simulink model "MIAC_ZTransform_PLC_Coder_not_external_Tustin_test"  (R2018b)
settings: Solver=FixedStepDiscrete  StartTime=0.0  StopTime=60000  FixedStep=1  RelTol=1e-3
libraries: simulink x4, slident x4
(part 1 of 2)
settings Model: Creator=Trips  LastModifiedBy=Trips
settings ConfigComp: PLC_OutputDir=PLCCoder  PLC_TargetIDE=step7  PLC_GenerateReport=off  PLC_LaunchReport=off

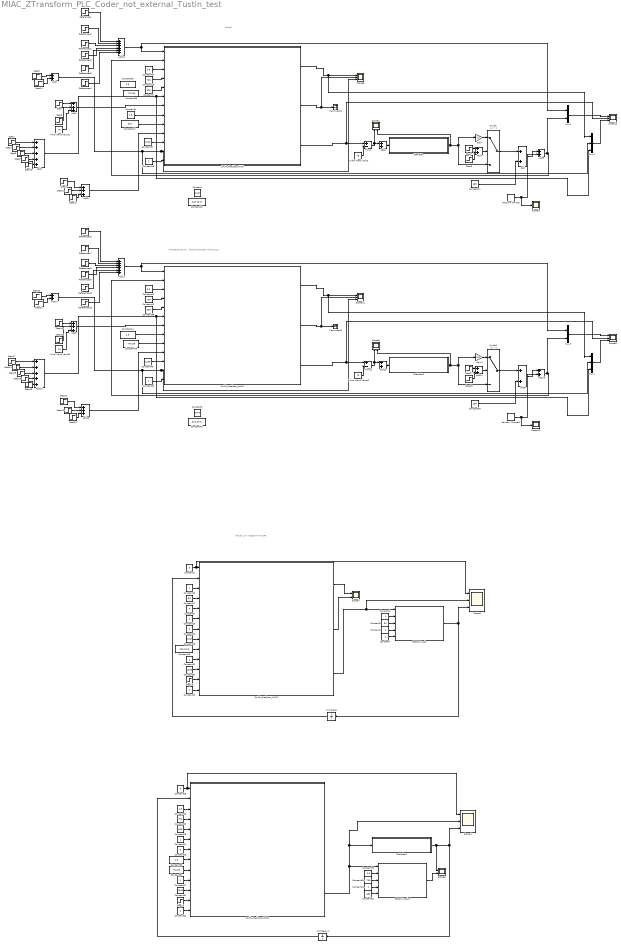
== system MIAC_ZTransform_PLC_Coder_not_external_Tustin_test ==
  note: Mit Adaptivem PI ...funktioniert aber nicht so gut
  note: Aktuell
  note: Aktuell zum vergleich mit SPS
  Add{,3..4,6..8,13..14,16..17} (10 alike) : Sum
  Add{1,5,9,15} (4 alike) : Sum  Inputs=+++
  Add10 : Sum  Inputs=++++++
  Add11 : Sum  Inputs=++++++
  Add12 : Sum  Inputs=5
  Add2 : Sum  Inputs=5
  Constant : Constant  Value=3.047
  Constant{1,28,32,38} (4 alike) : Constant  Value=600
  Constant{4,6,10,13,16,18,21..22,24,27,31,43} (12 alike) : Constant
  Constant11 : Constant  Value=165
  Constant12 : Constant  Value=222.22*3
  Constant{14,19,29,41} (4 alike) : Constant  Value=0.5
  Constant{15,23,30,42} (4 alike) : Constant  Value=700
  Constant17 : Constant  Value=50
  Constant2 : Constant  Value=3
  Constant20 : Constant  Value=0
  Constant25 : Constant  Value=3
  Constant26 : Constant  Value=0
  Constant3 : Constant  Value=5
  Constant33 : Constant  Value=2.5
  Constant34 : Constant  Value=776.39
  Constant35 : Constant  Value=2.5
  Constant36 : Constant  Value=776.39
  Constant{37,46,50..51} (4 alike) : Constant  Value=1200
  Constant39 : Constant  Value=165
  Constant40 : Constant  Value=222.22*3
  Constant44 : Constant  Value=2.5
  Constant45 : Constant  Value=776.39
  Constant47 : Constant  Value=937
  Constant48 : Constant  Value=3.047
  Constant49 : Constant  Value=222.22*3
  Constant5 : Constant  Value=50
  Constant7 : Constant  Value=4
  Constant8 : Constant  Value=1.8
  Constant9 : Constant  Value=3.047
  Drehofen : Subsystem
  Drehofen1 : Subsystem
  Drehofen2 : Subsystem
  FOPDT_Tustin : Subsystem  TreatAsAtomicUnit=on  SystemSampleTime=1
  FOPDT_Tustin1 : Subsystem  TreatAsAtomicUnit=on  SystemSampleTime=1
  Gain : Gain  Gain=1.5
  Gain1 : Gain  Gain=1.5
  Initial Hand Value{,1..3} (4 alike) : Constant  Value=75
  Minus : Sum  Inputs=+-
  Minus1 : Sum  Inputs=+-
  Mux1 : Mux  Inputs=2
  Mux2 : Mux  Inputs=3
  Mux3 : Mux  Inputs=2
  Mux4 : Mux  Inputs=3
  Random Number : RandomNumber  Variance=0.01  SampleTime=10
  Random Number1 : RandomNumber  Variance=0.01  SampleTime=10
  References : Step  After=3
  References1 : Step  Time=12000  After=2
  References10 : Step  Time=0  After=165
  References11 : Step  Time=40000  After=-7
  References2 : Step  Time=18000  After=3
  References3 : Step  Time=35000  After=3
  References4 : Step  Time=0  After=165
  References5 : Step  Time=40000  After=-7
  References6 : Step  After=3
  References7 : Step  Time=12000  After=2
  References8 : Step  Time=18000  After=3
  References9 : Step  Time=35000  After=3
  Scope{1,5,7..8} (4 alike) : Scope  NumInputPorts=2
  Scope10 : Scope
  Scope{2,4,6,9,11..12} (6 alike) : Scope  NumInputPorts=3
  Scope3 : Scope
  Smith_Predictor_MIAC : Subsystem  TreatAsAtomicUnit=on  SystemSampleTime=1
  Smith_Predictor_MIAC1 : Subsystem  TreatAsAtomicUnit=on  SystemSampleTime=1
  Smith_Predictor_MIAC2 : Subsystem  TreatAsAtomicUnit=on  SystemSampleTime=1
  Smith_Predictor_MIAC4 : Subsystem  TreatAsAtomicUnit=on  SystemSampleTime=1
  Step : Step  Time=300  After=5  SampleTime=0
  Step1 : Step  Time=4000  SampleTime=0
  Step10 : Step  Time=50000  SampleTime=0
  Step11 : Step  Time=35000  After=-1  SampleTime=0
  Step12 : Step  Time=38000  SampleTime=1
  Step13 : Step  Time=500  After=0  SampleTime=0
  Step14 : Step  Time=2.5*10^4  SampleTime=1
  Step15 : Step  Time=500  After=0  SampleTime=0
  Step16 : Step  Time=300  After=5  SampleTime=0
  Step17 : Step  Time=4000  SampleTime=0
  Step18 : Step  Time=50000  SampleTime=0
  Step19 : Step  Time=35000  After=-1  SampleTime=0
  Step2 : Step  Time=3900  SampleTime=1
  Step20 : Step  Time=38000  SampleTime=1
  Step21 : Step  Time=2.5*10^4  SampleTime=1
  Step22 : Step  Time=3900  SampleTime=1
  Step23 : Step  Time=5000  Before=1  After=0  SampleTime=1
  Step24 : Step  Time=20000  After=-1  SampleTime=0
  Step25 : Step  Time=25000  SampleTime=0
  Step26 : Step  Time=19000  After=5  SampleTime=0
  Step27 : Step  Time=3*10^4  SampleTime=0
  Step28 : Step  Time=3.8*10^4  After=0  SampleTime=0
  Step29 : Step  Time=45000  After=-1  SampleTime=0
  Step3 : Step  Time=5000  Before=1  After=0  SampleTime=1
  Step4 : Step  Time=20000  After=-1  SampleTime=0
  Step5 : Step  Time=25000  SampleTime=0
  Step6 : Step  Time=19000  After=5  SampleTime=0
  Step7 : Step  Time=3*10^4  SampleTime=0
  Step8 : Step  Time=3.8*10^4  After=0  SampleTime=0
  Step9 : Step  Time=45000  After=-1  SampleTime=0
  Switch : Switch  Criteria=u2 > Threshold
  Switch1 : Switch  Criteria=u2 > Threshold
  Terminator1 : Terminator
  Terminator2 : Terminator
  Unit Delay : UnitDelay  SampleTime=-1
  Unit Delay1 : UnitDelay  SampleTime=-1
  wires:
  Smith_Predictor_MIAC/1(Gain_NOT_Filtered) -> Mux2/1, Scope6/1  "Gain Filtered"
  Smith_Predictor_MIAC/2(Gain_Filtered) -> Scope6/2, Terminator1/1
  Add10/1 -> Mux1/1, Smith_Predictor_MIAC/1(Setpoint)  "setpoint"
  Step8/1 -> Add4/2
  Smith_Predictor_MIAC/3(Controller_Value) -> Scope12/2, Minus/1  "Adaptive"
  Add4/1 -> Switch/2  "Fehler ein"
  Gain/1 -> Switch/1
  Minus/1 -> Add6/1, Scope1/1
  Add6/1 -> Drehofen/1(In1)
  Drehofen/1(Out1) -> Scope1/2, Gain/1, Switch/3
  Step7/1 -> Add4/1
  Random Number/1 -> Scope3/1, Add3/2
  Initial Hand Value/1 -> Minus/2
  Add/1 -> Add3/1  "MIAC_SmithPredictor"
  Switch/1 -> Add/1  "MIAC_SmithPredictor"
  Constant11/1 -> Add/2
  Add3/1 -> Mux1/2, Smith_Predictor_MIAC/2(Process_Value)  "MIAC_SmithPredictor"
  References3/1 -> Add10/4  "r"
  References/1 -> Add10/1  "r"
  References4/1 -> Add10/6  "r"
  References1/1 -> Add10/2  "r"
  References2/1 -> Add10/3  "r"
  References5/1 -> Add10/5
  Constant8/1 -> Smith_Predictor_MIAC/8(P_Controller)
  Constant47/1 -> Smith_Predictor_MIAC/9(I_Controller)
  Constant14/1 -> Smith_Predictor_MIAC/3(Gain_System)
  Constant15/1 -> Smith_Predictor_MIAC/4(Time_Constant_System)
  Constant16/1 -> Smith_Predictor_MIAC/13(Sample_Time)
  Constant1/1 -> Smith_Predictor_MIAC/5(Dead_Time_System)
  Step14/1 -> Add7/2  "Start Adaption"
  Step3/1 -> Add7/1  "Start Adaption"
  Add7/1 -> Mux2/2, Scope6/3, Smith_Predictor_MIAC/12(Enable_Adaption)  "Start Adaption"
  Step6/1 -> Add1/2
  Initial Hand Value1/1 -> Add1/3
  Step/1 -> Add1/1
  Add1/1 -> Smith_Predictor_MIAC/7(Hand_Value)
  Step9/1 -> Add2/4  "Einschalten Automatik"
  Step10/1 -> Add2/5  "Einschalten Automatik"
  Step5/1 -> Add2/3  "Einschalten Automatik"
  Step4/1 -> Add2/2  "Einschalten Automatik"
  Step1/1 -> Add2/1  "Einschalten Automatik"
  Add2/1 -> Mux2/3, Smith_Predictor_MIAC/6(" Enable_Auto")  "Einschalten Automatik"
  Step12/1 -> Add5/3  "Start Identification"
  Step11/1 -> Add5/2  "Einschalten Automatik"
  Step2/1 -> Add5/1  "Start Identification"
  Add5/1 -> Smith_Predictor_MIAC/10(Start_Identification)  "Start Identification"
  Constant6/1 -> FOPDT_Tustin/4(Sample_Time)
  Constant17/1 -> Smith_Predictor_MIAC1/4(Time_Constant_System)
  Constant21/1 -> Smith_Predictor_MIAC1/10(Start_Identification)
  Constant10/1 -> Smith_Predictor_MIAC1/3(Gain_System)
  Constant49/1 -> Smith_Predictor_MIAC1/9(I_Controller)
  Constant18/1 -> Smith_Predictor_MIAC1/6(" Enable_Auto")
  Constant48/1 -> Smith_Predictor_MIAC1/8(P_Controller)
  Constant7/1 -> FOPDT_Tustin/5(" Dead_Time")
  Constant4/1 -> FOPDT_Tustin/2(Gain_System)
  Constant20/1 -> Smith_Predictor_MIAC1/7(Hand_Value)
  Constant2/1 -> Smith_Predictor_MIAC1/1(Setpoint), Scope2/1
  Constant5/1 -> FOPDT_Tustin/3(Time_Constant_System)
  Constant3/1 -> Smith_Predictor_MIAC1/5(Dead_Time_System)
  Smith_Predictor_MIAC1/3(Controller_Value) -> Scope2/2, FOPDT_Tustin/1(FOPD_Input)  "Adaptive"
  FOPDT_Tustin/1(FOPD_Output) -> Unit Delay/1, Scope2/3  "tustin"
  Unit Delay/1 -> Smith_Predictor_MIAC1/2(Process_Value)
  Unit Delay1/1 -> Smith_Predictor_MIAC2/2(Process_Value)
  Constant22/1 -> Smith_Predictor_MIAC2/13(Sample_Time)
  Drehofen1/1(Out1) -> Scope5/1, Scope4/3, Unit Delay1/1
  Constant26/1 -> Smith_Predictor_MIAC2/7(Hand_Value)
  Constant34/1 -> Smith_Predictor_MIAC2/9(I_Controller)
  Constant19/1 -> Smith_Predictor_MIAC2/3(Gain_System)
  Constant28/1 -> Smith_Predictor_MIAC2/5(Dead_Time_System)
  Constant33/1 -> Smith_Predictor_MIAC2/8(P_Controller)
  Constant27/1 -> Smith_Predictor_MIAC2/10(Start_Identification)
  Constant25/1 -> Smith_Predictor_MIAC2/1(Setpoint), Scope4/1
  Constant23/1 -> Smith_Predictor_MIAC2/4(Time_Constant_System)
  Constant24/1 -> Smith_Predictor_MIAC2/6(" Enable_Auto")
  Step15/1 -> Smith_Predictor_MIAC2/12(Enable_Adaption)
  Smith_Predictor_MIAC2/3(Controller_Value) -> FOPDT_Tustin1/1(FOPD_Input), Drehofen1/1(In1), Scope4/2  "Adaptive"
  Constant29/1 -> FOPDT_Tustin1/2(Gain_System)
  Constant31/1 -> FOPDT_Tustin1/4(Sample_Time)
  Constant30/1 -> FOPDT_Tustin1/3(Time_Constant_System)
  Constant32/1 -> FOPDT_Tustin1/5(" Dead_Time")
  FOPDT_Tustin1/1(FOPD_Output) -> Scope5/2  "tustin"
  Smith_Predictor_MIAC1/1(Gain_NOT_Filtered) -> Scope7/1  "Gain Filtered"
  Smith_Predictor_MIAC1/2(Gain_Filtered) -> Scope7/2
  Constant37/1 -> Smith_Predictor_MIAC/11(Time_Constant_Gain_identification_Filter)
  Mux1/1 -> Scope12/1
  Mux2/1 -> Scope12/3
  Mux3/1 -> Scope9/1
  Step20/1 -> Add15/3  "Start Identification"
  Step17/1 -> Add12/1  "Einschalten Automatik"
  Step25/1 -> Add12/3  "Einschalten Automatik"
  Step24/1 -> Add12/2  "Einschalten Automatik"
  References9/1 -> Add11/4  "r"
  Step19/1 -> Add15/2  "Einschalten Automatik"
  Step21/1 -> Add17/2  "Start Adaption"
  Step23/1 -> Add17/1  "Start Adaption"
  Add11/1 -> Mux3/1, Smith_Predictor_MIAC4/1(Setpoint)  "setpoint"
  References10/1 -> Add11/6  "r"
  Step29/1 -> Add12/4  "Einschalten Automatik"
  Add13/1 -> Mux3/2, Smith_Predictor_MIAC4/2(Process_Value)  "MIAC_SmithPredictor"
  Constant39/1 -> Add8/2
  Gain1/1 -> Switch1/1
  Random Number1/1 -> Scope10/1, Add13/2
  Initial Hand Value3/1 -> Add9/3
  Add16/1 -> Drehofen2/1(In1)
  Drehofen2/1(Out1) -> Scope8/2, Gain1/1, Switch1/3
  Step18/1 -> Add12/5  "Einschalten Automatik"
  Constant46/1 -> Smith_Predictor_MIAC4/11(Time_Constant_Gain_identification_Filter)
  Switch1/1 -> Add8/1  "MIAC_SmithPredictor"
  Constant43/1 -> Smith_Predictor_MIAC4/13(Sample_Time)
  Step28/1 -> Add14/2
  Smith_Predictor_MIAC4/2(Gain_Filtered) -> Scope11/2, Terminator2/1
  Constant44/1 -> Smith_Predictor_MIAC4/8(P_Controller)
  Step27/1 -> Add14/1
  Add15/1 -> Smith_Predictor_MIAC4/10(Start_Identification)  "Start Identification"
  Add17/1 -> Mux4/2, Scope11/3, Smith_Predictor_MIAC4/12(Enable_Adaption)  "Start Adaption"
  Constant45/1 -> Smith_Predictor_MIAC4/9(I_Controller)
  Mux4/1 -> Scope9/3
  Smith_Predictor_MIAC4/1(Gain_NOT_Filtered) -> Mux4/1, Scope11/1  "Gain Filtered"
  Initial Hand Value2/1 -> Minus1/2
  Add14/1 -> Switch1/2  "Fehler ein"
  Smith_Predictor_MIAC4/3(Controller_Value) -> Scope9/2, Minus1/1  "Adaptive"
  References11/1 -> Add11/5
  Constant41/1 -> Smith_Predictor_MIAC4/3(Gain_System)
  References7/1 -> Add11/2  "r"
  Add9/1 -> Smith_Predictor_MIAC4/7(Hand_Value)
  References6/1 -> Add11/1  "r"
  Step16/1 -> Add9/1
  Step22/1 -> Add15/1  "Start Identification"
  Add8/1 -> Add13/1  "MIAC_SmithPredictor"
  Add12/1 -> Mux4/3, Smith_Predictor_MIAC4/6(" Enable_Auto")  "Einschalten Automatik"
  Constant42/1 -> Smith_Predictor_MIAC4/4(Time_Constant_System)
  References8/1 -> Add11/3  "r"
  Minus1/1 -> Add16/1, Scope8/1
  Constant38/1 -> Smith_Predictor_MIAC4/5(Dead_Time_System)
  Step26/1 -> Add9/2
  Step13/1 -> Smith_Predictor_MIAC1/12(Enable_Adaption)
  Constant13/1 -> Smith_Predictor_MIAC1/13(Sample_Time)
  Constant50/1 -> Smith_Predictor_MIAC1/11(Time_Constant_Gain_identification_Filter)
  Constant51/1 -> Smith_Predictor_MIAC2/11(Time_Constant_Gain_identification_Filter)

== system MIAC_ZTransform_PLC_Coder_not_external_Tustin_test/Drehofen ==
  In1 : Inport
  Constant3 : Constant  Value=0.5/700
  Constant4 : Constant  Value=[1 -exp(-1/700)]
  Delay : Delay  DelayLength=600
  Discrete Transfer Fcn : DiscreteTransferFcn  NumeratorSource=Input port  DenominatorSource=Input port  a0EqualsOne=on
      settings: InputPortMap=u0,p1,p3
  Out1 : Outport
  wires:
  Discrete Transfer Fcn/1 -> Delay/1
  Constant4/1 -> Discrete Transfer Fcn/3
  Constant3/1 -> Discrete Transfer Fcn/2
  In1/1 -> Discrete Transfer Fcn/1
  Delay/1 -> Out1/1  "MIAC_SmithPredictor"

== system MIAC_ZTransform_PLC_Coder_not_external_Tustin_test/Drehofen1 ==
  In1 : Inport
  Constant3 : Constant  Value=0.5/700
  Constant4 : Constant  Value=[1 -exp(-1/700)]
  Delay : Delay  DelayLength=600
  Discrete Transfer Fcn : DiscreteTransferFcn  NumeratorSource=Input port  DenominatorSource=Input port  a0EqualsOne=on
      settings: InputPortMap=u0,p1,p3
  Out1 : Outport
  wires:
  Discrete Transfer Fcn/1 -> Delay/1
  Constant4/1 -> Discrete Transfer Fcn/3
  Constant3/1 -> Discrete Transfer Fcn/2
  In1/1 -> Discrete Transfer Fcn/1
  Delay/1 -> Out1/1  "MIAC_SmithPredictor"

== system MIAC_ZTransform_PLC_Coder_not_external_Tustin_test/Drehofen2 ==
  In1 : Inport
  Constant3 : Constant  Value=0.5/700
  Constant4 : Constant  Value=[1 -exp(-1/700)]
  Delay : Delay  DelayLength=600
  Discrete Transfer Fcn : DiscreteTransferFcn  NumeratorSource=Input port  DenominatorSource=Input port  a0EqualsOne=on
      settings: InputPortMap=u0,p1,p3
  Out1 : Outport
  wires:
  Discrete Transfer Fcn/1 -> Delay/1
  Constant4/1 -> Discrete Transfer Fcn/3
  Constant3/1 -> Discrete Transfer Fcn/2
  In1/1 -> Discrete Transfer Fcn/1
  Delay/1 -> Out1/1  "MIAC_SmithPredictor"

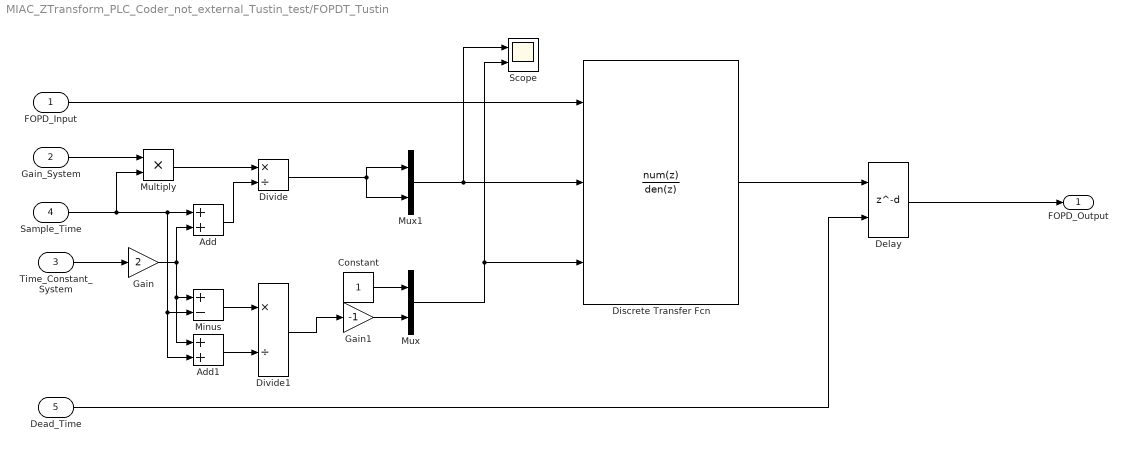
== system MIAC_ZTransform_PLC_Coder_not_external_Tustin_test/FOPDT_Tustin ==
  FOPD_Input : Inport
  Gain_System : Inport  Port=2
  Time_Constant_System : Inport  Port=3
  Sample_Time : Inport  Port=4
  " Dead_Time" : Inport  Port=5
  Add : Sum
  Add1 : Sum
  Constant : Constant
  Delay : Delay  DelayLengthSource=Input port  DelayLength=600  DelayLengthUpperLimit=800
      settings: InputPortMap=u0,p1
  Discrete Transfer Fcn : DiscreteTransferFcn  NumeratorSource=Input port  DenominatorSource=Input port  SampleTime=1  a0EqualsOne=on
      settings: InputPortMap=u0,p1,p3
  Divide : Product  Inputs=*/
  Divide1 : Product  Inputs=*/
  Gain : Gain  Gain=2
  Gain1 : Gain  Gain=-1
  Minus : Sum  Inputs=+-
  Multiply : Product
  Mux : Mux  Inputs=2
  Mux1 : Mux  Inputs=2
  Scope : Scope  NumInputPorts=2
  FOPD_Output : Outport
  wires:
  FOPD_Input/1 -> Discrete Transfer Fcn/1
  Discrete Transfer Fcn/1 -> Delay/1
  Mux/1 -> Scope/2, Discrete Transfer Fcn/3
  " Dead_Time"/1 -> Delay/2
  Sample_Time/1 -> Add1/2, Minus/2, Add/1, Multiply/2
  Mux1/1 -> Scope/1, Discrete Transfer Fcn/2
  Time_Constant_System/1 -> Gain/1
  Delay/1 -> FOPD_Output/1
  Gain_System/1 -> Multiply/1
  Multiply/1 -> Divide/1
  Gain/1 -> Add1/1, Minus/1, Add/2
  Add/1 -> Divide/2
  Divide/1 -> Mux1/2, Mux1/1
  Constant/1 -> Mux/1
  Minus/1 -> Divide1/1
  Add1/1 -> Divide1/2
  Divide1/1 -> Gain1/1
  Gain1/1 -> Mux/2

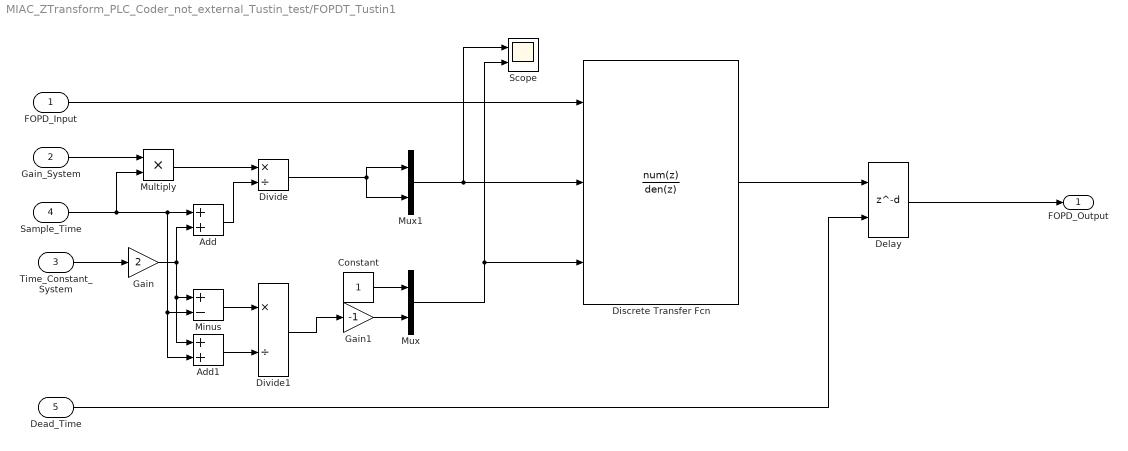
== system MIAC_ZTransform_PLC_Coder_not_external_Tustin_test/FOPDT_Tustin1 ==
  FOPD_Input : Inport
  Gain_System : Inport  Port=2
  Time_Constant_System : Inport  Port=3
  Sample_Time : Inport  Port=4
  " Dead_Time" : Inport  Port=5
  Add : Sum
  Add1 : Sum
  Constant : Constant
  Delay : Delay  DelayLengthSource=Input port  DelayLength=600  DelayLengthUpperLimit=800
      settings: InputPortMap=u0,p1
  Discrete Transfer Fcn : DiscreteTransferFcn  NumeratorSource=Input port  DenominatorSource=Input port  SampleTime=1  a0EqualsOne=on
      settings: InputPortMap=u0,p1,p3
  Divide : Product  Inputs=*/
  Divide1 : Product  Inputs=*/
  Gain : Gain  Gain=2
  Gain1 : Gain  Gain=-1
  Minus : Sum  Inputs=+-
  Multiply : Product
  Mux : Mux  Inputs=2
  Mux1 : Mux  Inputs=2
  Scope : Scope  NumInputPorts=2
  FOPD_Output : Outport
  wires:
  FOPD_Input/1 -> Discrete Transfer Fcn/1
  Discrete Transfer Fcn/1 -> Delay/1
  Mux/1 -> Scope/2, Discrete Transfer Fcn/3
  " Dead_Time"/1 -> Delay/2
  Sample_Time/1 -> Add1/2, Minus/2, Add/1, Multiply/2
  Mux1/1 -> Scope/1, Discrete Transfer Fcn/2
  Time_Constant_System/1 -> Gain/1
  Delay/1 -> FOPD_Output/1
  Gain_System/1 -> Multiply/1
  Multiply/1 -> Divide/1
  Gain/1 -> Add1/1, Minus/1, Add/2
  Add/1 -> Divide/2
  Divide/1 -> Mux1/2, Mux1/1
  Constant/1 -> Mux/1
  Minus/1 -> Divide1/1
  Add1/1 -> Divide1/2
  Divide1/1 -> Gain1/1
  Gain1/1 -> Mux/2

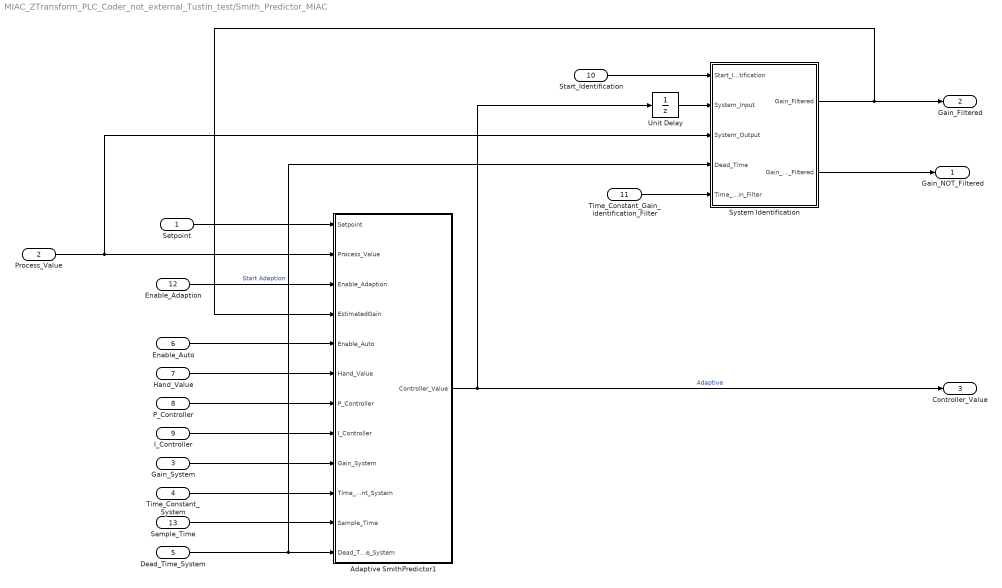
== system MIAC_ZTransform_PLC_Coder_not_external_Tustin_test/Smith_Predictor_MIAC ==
  Setpoint : Inport
  Process_Value : Inport  Port=2
  Gain_System : Inport  Port=3
  Time_Constant_System : Inport  Port=4
  Dead_Time_System : Inport  Port=5
  " Enable_Auto" : Inport  Port=6
  Hand_Value : Inport  Port=7
  P_Controller : Inport  Port=8
  I_Controller : Inport  Port=9
  Start_Identification : Inport  Port=10  PortDimensions=1  SampleTime=1
  Time_Constant_Gain_identification_Filter : Inport  Port=11
  Enable_Adaption : Inport  Port=12
  Sample_Time : Inport  Port=13
  Adaptive SmithPredictor1 : Subsystem  TreatAsAtomicUnit=on  SystemSampleTime=1
  System Identification : Subsystem  TreatAsAtomicUnit=on  SystemSampleTime=1
  Unit Delay : UnitDelay
  Gain_NOT_Filtered : Outport
  Gain_Filtered : Outport  Port=2
  Controller_Value : Outport  Port=3
  wires:
  Gain_System/1 -> Adaptive SmithPredictor1/9(Gain_System)
  Dead_Time_System/1 -> Adaptive SmithPredictor1/12(" Dead_Time_System"), System Identification/4(Dead_Time)
  Adaptive SmithPredictor1/1(Controller_Value) -> Unit Delay/1, Controller_Value/1  "Adaptive"
  Time_Constant_System/1 -> Adaptive SmithPredictor1/10(Time_Constant_System)
  P_Controller/1 -> Adaptive SmithPredictor1/7(P_Controller)
  Sample_Time/1 -> Adaptive SmithPredictor1/11(Sample_Time)
  I_Controller/1 -> Adaptive SmithPredictor1/8(I_Controller)
  Enable_Adaption/1 -> Adaptive SmithPredictor1/3(Enable_Adaption)  "Start Adaption"
  System Identification/2(Gain_Not_Filtered) -> Gain_NOT_Filtered/1
  Setpoint/1 -> Adaptive SmithPredictor1/1(Setpoint)
  Start_Identification/1 -> System Identification/1(Start_Identification)
  System Identification/1(Gain_Filtered) -> Gain_Filtered/1, Adaptive SmithPredictor1/4(EstimatedGain)
  " Enable_Auto"/1 -> Adaptive SmithPredictor1/5(Enable_Auto)
  Hand_Value/1 -> Adaptive SmithPredictor1/6(Hand_Value)
  Process_Value/1 -> System Identification/3(System_Output), Adaptive SmithPredictor1/2(Process_Value)
  Unit Delay/1 -> System Identification/2(System_Input)
  Time_Constant_Gain_identification_Filter/1 -> System Identification/5(Time_Constant_Gain_Filter)

== system MIAC_ZTransform_PLC_Coder_not_external_Tustin_test/Smith_Predictor_MIAC1 ==
  Setpoint : Inport
  Process_Value : Inport  Port=2
  Gain_System : Inport  Port=3
  Time_Constant_System : Inport  Port=4
  Dead_Time_System : Inport  Port=5
  " Enable_Auto" : Inport  Port=6
  Hand_Value : Inport  Port=7
  P_Controller : Inport  Port=8
  I_Controller : Inport  Port=9
  Start_Identification : Inport  Port=10  PortDimensions=1  SampleTime=1
  Time_Constant_Gain_identification_Filter : Inport  Port=11
  Enable_Adaption : Inport  Port=12
  Sample_Time : Inport  Port=13
  Adaptive SmithPredictor1 : Subsystem  TreatAsAtomicUnit=on  SystemSampleTime=1
  System Identification : Subsystem  TreatAsAtomicUnit=on  SystemSampleTime=1
  Unit Delay : UnitDelay
  Gain_NOT_Filtered : Outport
  Gain_Filtered : Outport  Port=2
  Controller_Value : Outport  Port=3
  wires:
  Gain_System/1 -> Adaptive SmithPredictor1/9(Gain_System)
  Dead_Time_System/1 -> Adaptive SmithPredictor1/12(" Dead_Time_System"), System Identification/4(Dead_Time)
  Adaptive SmithPredictor1/1(Controller_Value) -> Unit Delay/1, Controller_Value/1  "Adaptive"
  Time_Constant_System/1 -> Adaptive SmithPredictor1/10(Time_Constant_System)
  P_Controller/1 -> Adaptive SmithPredictor1/7(P_Controller)
  Sample_Time/1 -> Adaptive SmithPredictor1/11(Sample_Time)
  I_Controller/1 -> Adaptive SmithPredictor1/8(I_Controller)
  Enable_Adaption/1 -> Adaptive SmithPredictor1/3(Enable_Adaption)  "Start Adaption"
  System Identification/2(Gain_Not_Filtered) -> Gain_NOT_Filtered/1
  Setpoint/1 -> Adaptive SmithPredictor1/1(Setpoint)
  Start_Identification/1 -> System Identification/1(Start_Identification)
  System Identification/1(Gain_Filtered) -> Gain_Filtered/1, Adaptive SmithPredictor1/4(EstimatedGain)
  " Enable_Auto"/1 -> Adaptive SmithPredictor1/5(Enable_Auto)
  Hand_Value/1 -> Adaptive SmithPredictor1/6(Hand_Value)
  Process_Value/1 -> System Identification/3(System_Output), Adaptive SmithPredictor1/2(Process_Value)
  Unit Delay/1 -> System Identification/2(System_Input)
  Time_Constant_Gain_identification_Filter/1 -> System Identification/5(Time_Constant_Gain_Filter)

== system MIAC_ZTransform_PLC_Coder_not_external_Tustin_test/Smith_Predictor_MIAC2 ==
  Setpoint : Inport
  Process_Value : Inport  Port=2
  Gain_System : Inport  Port=3
  Time_Constant_System : Inport  Port=4
  Dead_Time_System : Inport  Port=5
  " Enable_Auto" : Inport  Port=6
  Hand_Value : Inport  Port=7
  P_Controller : Inport  Port=8
  I_Controller : Inport  Port=9
  Start_Identification : Inport  Port=10  PortDimensions=1  SampleTime=1
  Time_Constant_Gain_identification_Filter : Inport  Port=11
  Enable_Adaption : Inport  Port=12
  Sample_Time : Inport  Port=13
  Adaptive SmithPredictor1 : Subsystem  TreatAsAtomicUnit=on  SystemSampleTime=1
  System Identification : Subsystem  TreatAsAtomicUnit=on  SystemSampleTime=1
  Unit Delay : UnitDelay
  Gain_NOT_Filtered : Outport
  Gain_Filtered : Outport  Port=2
  Controller_Value : Outport  Port=3
  wires:
  Gain_System/1 -> Adaptive SmithPredictor1/9(Gain_System)
  Dead_Time_System/1 -> Adaptive SmithPredictor1/12(" Dead_Time_System"), System Identification/4(Dead_Time)
  Adaptive SmithPredictor1/1(Controller_Value) -> Unit Delay/1, Controller_Value/1  "Adaptive"
  Time_Constant_System/1 -> Adaptive SmithPredictor1/10(Time_Constant_System)
  P_Controller/1 -> Adaptive SmithPredictor1/7(P_Controller)
  Sample_Time/1 -> Adaptive SmithPredictor1/11(Sample_Time)
  I_Controller/1 -> Adaptive SmithPredictor1/8(I_Controller)
  Enable_Adaption/1 -> Adaptive SmithPredictor1/3(Enable_Adaption)  "Start Adaption"
  System Identification/2(Gain_Not_Filtered) -> Gain_NOT_Filtered/1
  Setpoint/1 -> Adaptive SmithPredictor1/1(Setpoint)
  Start_Identification/1 -> System Identification/1(Start_Identification)
  System Identification/1(Gain_Filtered) -> Gain_Filtered/1, Adaptive SmithPredictor1/4(EstimatedGain)
  " Enable_Auto"/1 -> Adaptive SmithPredictor1/5(Enable_Auto)
  Hand_Value/1 -> Adaptive SmithPredictor1/6(Hand_Value)
  Process_Value/1 -> System Identification/3(System_Output), Adaptive SmithPredictor1/2(Process_Value)
  Unit Delay/1 -> System Identification/2(System_Input)
  Time_Constant_Gain_identification_Filter/1 -> System Identification/5(Time_Constant_Gain_Filter)

== system MIAC_ZTransform_PLC_Coder_not_external_Tustin_test/Smith_Predictor_MIAC4 ==
  Setpoint : Inport
  Process_Value : Inport  Port=2
  Gain_System : Inport  Port=3
  Time_Constant_System : Inport  Port=4
  Dead_Time_System : Inport  Port=5
  " Enable_Auto" : Inport  Port=6
  Hand_Value : Inport  Port=7
  P_Controller : Inport  Port=8
  I_Controller : Inport  Port=9
  Start_Identification : Inport  Port=10  PortDimensions=1  SampleTime=1
  Time_Constant_Gain_identification_Filter : Inport  Port=11
  Enable_Adaption : Inport  Port=12
  Sample_Time : Inport  Port=13
  Adaptive SmithPredictor1 : Subsystem  TreatAsAtomicUnit=on  SystemSampleTime=1
  System Identification : Subsystem  TreatAsAtomicUnit=on  SystemSampleTime=1
  Unit Delay : UnitDelay
  Gain_NOT_Filtered : Outport
  Gain_Filtered : Outport  Port=2
  Controller_Value : Outport  Port=3
  wires:
  Gain_System/1 -> Adaptive SmithPredictor1/9(Gain_System)
  Dead_Time_System/1 -> Adaptive SmithPredictor1/12(" Dead_Time_System"), System Identification/4(Dead_Time)
  Adaptive SmithPredictor1/1(Controller_Value) -> Unit Delay/1, Controller_Value/1  "Adaptive"
  Time_Constant_System/1 -> Adaptive SmithPredictor1/10(Time_Constant_System)
  P_Controller/1 -> Adaptive SmithPredictor1/7(P_Controller)
  Sample_Time/1 -> Adaptive SmithPredictor1/11(Sample_Time)
  I_Controller/1 -> Adaptive SmithPredictor1/8(I_Controller)
  Enable_Adaption/1 -> Adaptive SmithPredictor1/3(Enable_Adaption)  "Start Adaption"
  System Identification/2(Gain_Not_Filtered) -> Gain_NOT_Filtered/1
  Setpoint/1 -> Adaptive SmithPredictor1/1(Setpoint)
  Start_Identification/1 -> System Identification/1(Start_Identification)
  System Identification/1(Gain_Filtered) -> Gain_Filtered/1, Adaptive SmithPredictor1/4(EstimatedGain)
  " Enable_Auto"/1 -> Adaptive SmithPredictor1/5(Enable_Auto)
  Hand_Value/1 -> Adaptive SmithPredictor1/6(Hand_Value)
  Process_Value/1 -> System Identification/3(System_Output), Adaptive SmithPredictor1/2(Process_Value)
  Unit Delay/1 -> System Identification/2(System_Input)
  Time_Constant_Gain_identification_Filter/1 -> System Identification/5(Time_Constant_Gain_Filter)

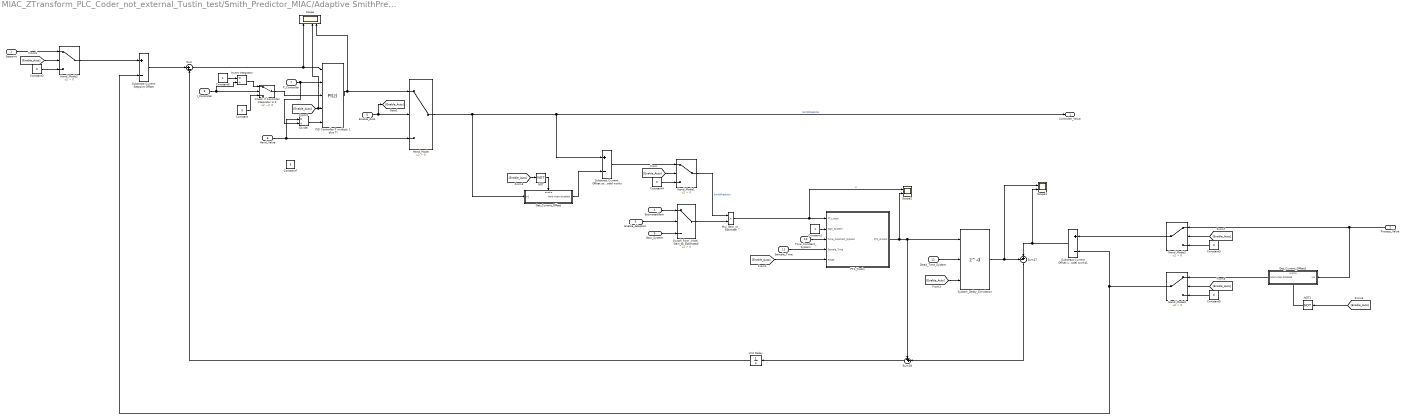
== system MIAC_ZTransform_PLC_Coder_not_external_Tustin_test/Smith_Predictor_MIAC/Adaptive SmithPredictor1 ==
  Setpoint : Inport
  Process_Value : Inport  Port=2
  Enable_Adaption : Inport  Port=3
  EstimatedGain : Inport  Port=4
  Enable_Auto : Inport  Port=5
  Hand_Value : Inport  Port=6
  P_Controller : Inport  Port=7
  I_Controller : Inport  Port=8
  Gain_System : Inport  Port=9
  Time_Constant_System : Inport  Port=10
  Sample_Time : Inport  Port=11
  " Dead_Time_System" : Inport  Port=12
  Check if Controller Integrator is 0 : Switch  Criteria=u2 ~= 0
  Constant{,2..5} (5 alike) : Constant  Value=0
  Constant1 : Constant
  Constant6 : Constant
  Constant7 : Constant  Value=6
  Divide : Product  Inputs=*/
  Get_Current_Offset : Subsystem
  Get_Current_Offset1 : Subsystem
  Hand_Mode{,1..4} (5 alike) : Switch  Criteria=u2 > Threshold
  Invert Integrator : Product  Inputs=*/
  Mul_Gain_or_Estimate : Product
  NOT : Logic  Operator=NOT  IconShape=distinctive  AllPortsSameDT=off  OutDataTypeStr=boolean
  NOT1 : Logic  Operator=NOT  IconShape=distinctive  AllPortsSameDT=off  OutDataTypeStr=boolean
  "PID Controller P multiply 1 plus Ti " : simulink/Continuous/PID Controller  Controller=PI  Form=Ideal  TimeDomain=Discrete-time  SampleTime=1  IntegratorMethod=Forward Euler  FilterMethod=Forward Euler  ControllerParametersSource=external  P=3.04732259067536  I=0.00445689106465138  D=118.272348286844  UseFilter=on  N=0.00420306193364532  TunerSelectOption=Transfer Function Based (PID Tuner App)  InitialConditionSource=external  InitialConditionForIntegrator=0  InitialConditionForFilter=0  DifferentiatorICPrevScaledInput=0  ExternalReset=rising  TrackingMode=off  Kt=1  LimitOutput=on  UpperSaturationLimit=100  LowerSaturationLimit=0  LinearizeAsGain=on  AntiWindupMode=none  Kb=1  POutMin=[]  POutMax=[]  IOutMin=[]  IOutMax=[]  DOutMin=[]  DOutMax=[]  NOutMin=[]  NOutMax=[]  SumOutMin=[]  SumOutMax=[]  SaturationOutMin=[]  SaturationOutMax=[]  PParamMin=[]  PParamMax=[]  IParamMin=[]  IParamMax=[]  DParamMin=[]  DParamMax=[]  NParamMin=[]  NParamMax=[]  KbParamMin=[]  KbParamMax=[]  KtParamMin=[]  KtParamMax=[]  KbOutMin=[]  KbOutMax=[]  KtOutMin=[]  KtOutMax=[]  IntegratorOutMin=[]  IntegratorOutMax=[]  FilterOutMin=[]  FilterOutMax=[]  SumI1OutMin=[]  SumI1OutMax=[]  SumI2OutMin=[]  SumI2OutMax=[]  SumI3OutMin=[]  SumI3OutMax=[]  SumI4OutMin=[]  SumI4OutMax=[]  SumDOutMin=[]  SumDOutMax=[]  DifferentiatorOutMin=[]  DifferentiatorOutMax=[]  FilterDiffOutCoefMin=[]  FilterDiffOutCoefMax=[]  ReciprocalOutMin=[]  ReciprocalOutMax=[]  SumDenOutMin=[]  SumDenOutMax=[]  SumNumOutMin=[]  SumNumOutMax=[]  DivideOutMin=[]  DivideOutMax=[]  IntegratorContinuousStateAttributes=''  IntegratorStateMustResolveToSignalObject=off  IntegratorRTWStateStorageClass=Auto  FilterContinuousStateAttributes=''  FilterStateMustResolveToSignalObject=off  FilterRTWStateStorageClass=Auto  ParallelPVariant=Passthrough  IdealPVariant=ExternalParameters  IVariant=ExternalParameters  DVariant=Disabled  IntegratorVariant=Discrete  SatVariant=Enabled  AWVariant=Passthrough  PCopyVariant=Disabled  TRVariant=Disabled  FdbkBlocksVariant=Forward  IdealPFdbkVariant=Disabled  SatFdbkVariant=Disabled  DerivativeFilterVariant=Disabled  NVariant=Disabled  NCopyVariant=Disabled_SignalSpec  FilterICVariant=Disabled  IntegratorICVariant=ExternalICs  ExternalResetVariant=ExternalReset  TRSumVariant=Passthrough  SumFdbkVariant=Disabled  SumVariant=Sum_PI
  PT1_Tustin : Subsystem  TreatAsAtomicUnit=on  SystemSampleTime=1
  Scope : Scope  NumInputPorts=4
  Scope1 : Scope  NumInputPorts=2
  Scope2 : Scope  NumInputPorts=2
  Substract Current Offset so that the linearised model works : Sum  Inputs=+-
  Substract Current Offset so that the linearised model works1 : Sum  Inputs=+-
  Substract Current Setpoint Offset : Sum  Inputs=+-
  Sum : Sum  Inputs=|+-
  Sum17 : Sum  Inputs=-+|
  Sum18 : Sum  Inputs=++|
  Switch_from_initial_Gain_to_Estimated : Switch  Criteria=u2 > Threshold
  System_Delay_Simulation : Delay  DelayLengthSource=Input port  DelayLength=600  DelayLengthUpperLimit=800  ExternalReset=Rising  SampleTime=1
      settings: InputPortMap=u0,p1,r5
  Unit Delay : UnitDelay
  Controller_Value : Outport
  wires:
  Substract Current Setpoint Offset/1 -> Sum/1
  Sum/1 -> "PID Controller P multiply 1 plus Ti "/1, Scope/1
  Hand_Mode/1 -> Get_Current_Offset/1(In1), Controller_Value/1, Substract Current Offset so that the linearised model works/1  "SmithPredictor"
  Substract Current Offset so that the linearised model works1/1 -> Scope1/2, Sum17/2
  PT1_Tustin/1(PT1_Output) -> Scope2/2, Sum18/1, System_Delay_Simulation/1
  System_Delay_Simulation/1 -> Scope1/1, Sum17/1
  Sum17/1 -> Sum18/2
  Mul_Gain_or_Estimate/1 -> Scope2/1, PT1_Tustin/1(PT1_Input)  "U"
  Switch_from_initial_Gain_to_Estimated/1 -> Mul_Gain_or_Estimate/2
  "PID Controller P multiply 1 plus Ti "/1 -> Hand_Mode/1, Scope/4
  Hand_Value/1 -> Divide/1, Hand_Mode/3
  Enable_Auto/1 -> [Enable_Auto], Hand_Mode/2
  P_Controller/1 -> Divide/2, "PID Controller P multiply 1 plus Ti "/2
  Check if Controller Integrator is 0/1 -> "PID Controller P multiply 1 plus Ti "/3
  " Dead_Time_System"/1 -> System_Delay_Simulation/2
  Gain_System/1 -> Switch_from_initial_Gain_to_Estimated/3
  Enable_Adaption/1 -> Switch_from_initial_Gain_to_Estimated/2
  EstimatedGain/1 -> Switch_from_initial_Gain_to_Estimated/1
  [Enable_Auto] -> Hand_Mode1/2
  Hand_Mode1/1 -> Mul_Gain_or_Estimate/1  "SmithPredictor"
  Constant4/1 -> Hand_Mode1/3
  [Enable_Auto] -> PT1_Tustin/5(Reset)
  [Enable_Auto] -> System_Delay_Simulation/3
  Substract Current Offset so that the linearised model works/1 -> Hand_Mode1/1
  Get_Current_Offset/1(Hold when disabled) -> Substract Current Offset so that the linearised model works/2
  [Enable_Auto] -> NOT/1
  NOT/1 -> Get_Current_Offset/Enable
  Sum18/1 -> Unit Delay/1
  Hand_Mode2/1 -> Substract Current Setpoint Offset/1
  NOT1/1 -> Get_Current_Offset1/Enable
  [Enable_Auto] -> NOT1/1
  Hand_Mode4/1 -> Substract Current Setpoint Offset/2, Substract Current Offset so that the linearised model works1/2
  Setpoint/1 -> Hand_Mode2/1
  [Enable_Auto] -> Hand_Mode2/2
  Constant2/1 -> Hand_Mode2/3
  Process_Value/1 -> Get_Current_Offset1/1(In1), Hand_Mode3/1
  [Enable_Auto] -> Hand_Mode3/2
  Constant3/1 -> Hand_Mode3/3
  Hand_Mode3/1 -> Substract Current Offset so that the linearised model works1/1
  Constant5/1 -> Hand_Mode4/3
  [Enable_Auto] -> Hand_Mode4/2
  Get_Current_Offset1/1(Hold when disabled) -> Hand_Mode4/1
  Time_Constant_System/1 -> PT1_Tustin/3(Time_Constant_System)
  Constant1/1 -> PT1_Tustin/2(Gain_System)
  Sample_Time/1 -> PT1_Tustin/4(Sample_Time)
  I_Controller/1 -> Check if Controller Integrator is 0/2, Invert Integrator/2
  Constant/1 -> Check if Controller Integrator is 0/3
  Invert Integrator/1 -> Check if Controller Integrator is 0/1
  Constant6/1 -> Invert Integrator/1
  Unit Delay/1 -> Sum/2
  [Enable_Auto] -> Scope/3, "PID Controller P multiply 1 plus Ti "/4
  Divide/1 -> "PID Controller P multiply 1 plus Ti "/5

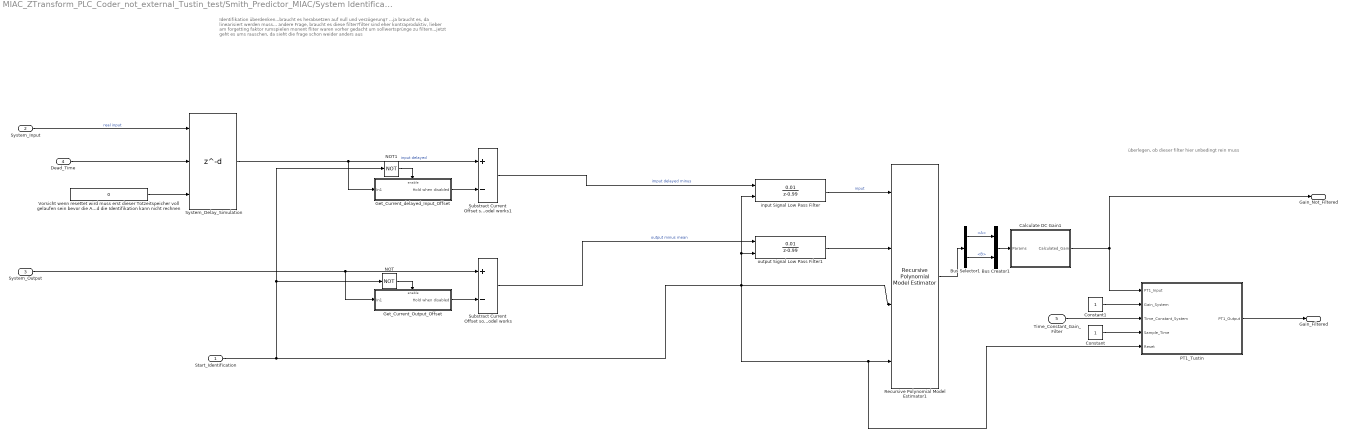
== system MIAC_ZTransform_PLC_Coder_not_external_Tustin_test/Smith_Predictor_MIAC/System Identification ==
  note: überlegen, ob dieser filter hier unbedingt rein muss
  note: Identifikation überdenken...braucht es herabsetzen auf null und verzögerung?
      | ...ja braucht es, da linearisiert werden muss...
      |
      | andere Frage, braucht es diese filter?filter sind eher kontraproduktiv, lieber am forgetting faktor rumspielen
      | monent fliter waren vorher gedacht um sollwertsprünge zu filtern...jetzt geht es ums rauschen, da sieht die frage schon weider anders aus
  Start_Identification : Inport  SampleTime=1
  System_Input : Inport  Port=2
  System_Output : Inport  Port=3  SampleTime=1
  Dead_Time : Inport  Port=4
  Time_Constant_Gain_Filter : Inport  Port=5
  Bus Creator1 : BusCreator  Inputs=2
  Bus Selector1 : BusSelector  OutputSignals=A,B
  Calculate DC Gain1 : Subsystem  TreatAsAtomicUnit=on  SystemSampleTime=1
  Constant : Constant
  Constant1 : Constant
  Get_Current_Output_Offset : Subsystem
  Get_Current_delayed_Input_Offset : Subsystem
  NOT : Logic  Operator=NOT  IconShape=distinctive  AllPortsSameDT=off  OutDataTypeStr=boolean
  NOT1 : Logic  Operator=NOT  IconShape=distinctive  AllPortsSameDT=off  OutDataTypeStr=boolean
  PT1_Tustin : Subsystem  TreatAsAtomicUnit=on  SystemSampleTime=1
  Recursive Polynomial Model Estimator1 : slident/Estimators/Recursive Polynomial Model Estimator  ModelStructure=ARX  InitialEstimateSource=None  A0=2  B0=1  C0=1  D0=1  F0=1  nk=1  P0=10  InitialInputs=0  InitialOutputs=0  History=Infinite  WindowLength=2000  EstimationMethod=Forgetting Factor  AdaptationParameter=1  HasTimeVaryingAdaptationParameter=off  NormalizationBias=eps  OutputError=off  OutputP=off  AddEnablePort=on  ExternalReset=Rising  InputProcessing=Sample-based  Ts=1
      settings: SourceProductName=System Identification Toolbox  SourceProductBaseCode=ID
  Substract Current Offset so that the linearised model works : Sum  Inputs=+-
  Substract Current Offset so that the linearised model works1 : Sum  Inputs=+-
  System_Delay_Simulation : Delay  DelayLengthSource=Input port  DelayLength=600  DelayLengthUpperLimit=800  ExternalReset=Rising  SampleTime=1
      settings: InputPortMap=u0,p1,r5
  Vorsicht wenn resettet wird muss erst dieser Totzeitspeicher voll gelaufen sein bevor die Adaption starten darf Sonst kommt heir immer 0 raus und die Identifikation kann nicht rechnen : Constant  Value=0
  input Signal Low Pass Filter : DiscreteTransferFcn  Numerator=[0.01]  Denominator=[1 -0.99]  ExternalReset=Rising  SampleTime=1  a0EqualsOne=on
      settings: InputPortMap=u0,r7
  output Signal Low Pass Filter1 : DiscreteTransferFcn  Numerator=[0.01]  Denominator=[1 -0.99]  ExternalReset=Rising  SampleTime=1  a0EqualsOne=on
      settings: InputPortMap=u0,r7
  Gain_Filtered : Outport
  Gain_Not_Filtered : Outport  Port=2
  wires:
  Recursive Polynomial Model Estimator1/1 -> Bus Selector1/1
  input Signal Low Pass Filter/1 -> Recursive Polynomial Model Estimator1/1  "input"
  Bus Creator1/1 -> Calculate DC Gain1/1(Params)
  Bus Selector1/1 -> Bus Creator1/1  "<A>"
  Bus Selector1/2 -> Bus Creator1/2  "<B>"
  Substract Current Offset so that the linearised model works/1 -> output Signal Low Pass Filter1/1  "output minus mean"
  NOT/1 -> Get_Current_Output_Offset/Enable
  Get_Current_Output_Offset/1(Hold when disabled) -> Substract Current Offset so that the linearised model works/2
  System_Output/1 -> Get_Current_Output_Offset/1(In1), Substract Current Offset so that the linearised model works/1
  Get_Current_delayed_Input_Offset/1(Hold when disabled) -> Substract Current Offset so that the linearised model works1/2
  NOT1/1 -> Get_Current_delayed_Input_Offset/Enable
  PT1_Tustin/1(PT1_Output) -> Gain_Filtered/1
  System_Input/1 -> System_Delay_Simulation/1  "real input"
  Vorsicht wenn resettet wird muss erst dieser Totzeitspeicher voll gelaufen sein bevor die Adaption starten darf Sonst kommt heir immer 0 raus und die Identifikation kann nicht rechnen/1 -> System_Delay_Simulation/3
  Dead_Time/1 -> System_Delay_Simulation/2
  Substract Current Offset so that the linearised model works1/1 -> input Signal Low Pass Filter/1  "imput delayed minus"
  System_Delay_Simulation/1 -> Substract Current Offset so that the linearised model works1/1, Get_Current_delayed_Input_Offset/1(In1)  "input delayed"
  Calculate DC Gain1/1(Calculated_Gain) -> PT1_Tustin/1(PT1_Input), Gain_Not_Filtered/1
  Start_Identification/1 -> NOT/1, NOT1/1, PT1_Tustin/5(Reset), Recursive Polynomial Model Estimator1/4, output Signal Low Pass Filter1/2, input Signal Low Pass Filter/2, Recursive Polynomial Model Estimator1/3
  output Signal Low Pass Filter1/1 -> Recursive Polynomial Model Estimator1/2
  Constant/1 -> PT1_Tustin/4(Sample_Time)
  Constant1/1 -> PT1_Tustin/2(Gain_System)
  Time_Constant_Gain_Filter/1 -> PT1_Tustin/3(Time_Constant_System)

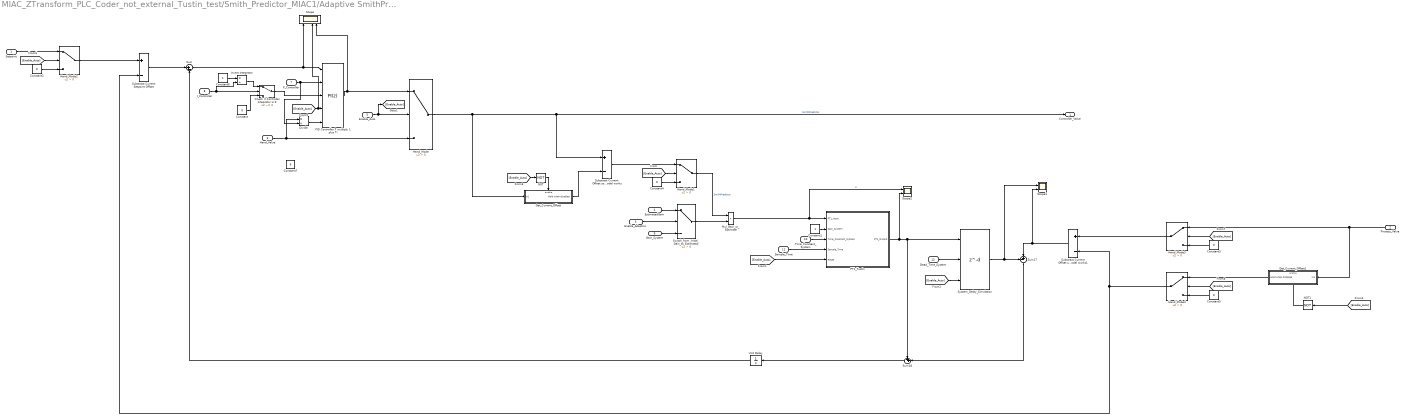
== system MIAC_ZTransform_PLC_Coder_not_external_Tustin_test/Smith_Predictor_MIAC1/Adaptive SmithPredictor1 ==
  Setpoint : Inport
  Process_Value : Inport  Port=2
  Enable_Adaption : Inport  Port=3
  EstimatedGain : Inport  Port=4
  Enable_Auto : Inport  Port=5
  Hand_Value : Inport  Port=6
  P_Controller : Inport  Port=7
  I_Controller : Inport  Port=8
  Gain_System : Inport  Port=9
  Time_Constant_System : Inport  Port=10
  Sample_Time : Inport  Port=11
  " Dead_Time_System" : Inport  Port=12
  Check if Controller Integrator is 0 : Switch  Criteria=u2 ~= 0
  Constant{,2..5} (5 alike) : Constant  Value=0
  Constant1 : Constant
  Constant6 : Constant
  Constant7 : Constant  Value=6
  Divide : Product  Inputs=*/
  Get_Current_Offset : Subsystem
  Get_Current_Offset1 : Subsystem
  Hand_Mode{,1..4} (5 alike) : Switch  Criteria=u2 > Threshold
  Invert Integrator : Product  Inputs=*/
  Mul_Gain_or_Estimate : Product
  NOT : Logic  Operator=NOT  IconShape=distinctive  AllPortsSameDT=off  OutDataTypeStr=boolean
  NOT1 : Logic  Operator=NOT  IconShape=distinctive  AllPortsSameDT=off  OutDataTypeStr=boolean
  "PID Controller P multiply 1 plus Ti " : simulink/Continuous/PID Controller  Controller=PI  Form=Ideal  TimeDomain=Discrete-time  SampleTime=1  IntegratorMethod=Forward Euler  FilterMethod=Forward Euler  ControllerParametersSource=external  P=3.04732259067536  I=0.00445689106465138  D=118.272348286844  UseFilter=on  N=0.00420306193364532  TunerSelectOption=Transfer Function Based (PID Tuner App)  InitialConditionSource=external  InitialConditionForIntegrator=0  InitialConditionForFilter=0  DifferentiatorICPrevScaledInput=0  ExternalReset=rising  TrackingMode=off  Kt=1  LimitOutput=on  UpperSaturationLimit=100  LowerSaturationLimit=0  LinearizeAsGain=on  AntiWindupMode=none  Kb=1  POutMin=[]  POutMax=[]  IOutMin=[]  IOutMax=[]  DOutMin=[]  DOutMax=[]  NOutMin=[]  NOutMax=[]  SumOutMin=[]  SumOutMax=[]  SaturationOutMin=[]  SaturationOutMax=[]  PParamMin=[]  PParamMax=[]  IParamMin=[]  IParamMax=[]  DParamMin=[]  DParamMax=[]  NParamMin=[]  NParamMax=[]  KbParamMin=[]  KbParamMax=[]  KtParamMin=[]  KtParamMax=[]  KbOutMin=[]  KbOutMax=[]  KtOutMin=[]  KtOutMax=[]  IntegratorOutMin=[]  IntegratorOutMax=[]  FilterOutMin=[]  FilterOutMax=[]  SumI1OutMin=[]  SumI1OutMax=[]  SumI2OutMin=[]  SumI2OutMax=[]  SumI3OutMin=[]  SumI3OutMax=[]  SumI4OutMin=[]  SumI4OutMax=[]  SumDOutMin=[]  SumDOutMax=[]  DifferentiatorOutMin=[]  DifferentiatorOutMax=[]  FilterDiffOutCoefMin=[]  FilterDiffOutCoefMax=[]  ReciprocalOutMin=[]  ReciprocalOutMax=[]  SumDenOutMin=[]  SumDenOutMax=[]  SumNumOutMin=[]  SumNumOutMax=[]  DivideOutMin=[]  DivideOutMax=[]  IntegratorContinuousStateAttributes=''  IntegratorStateMustResolveToSignalObject=off  IntegratorRTWStateStorageClass=Auto  FilterContinuousStateAttributes=''  FilterStateMustResolveToSignalObject=off  FilterRTWStateStorageClass=Auto  ParallelPVariant=Passthrough  IdealPVariant=ExternalParameters  IVariant=ExternalParameters  DVariant=Disabled  IntegratorVariant=Discrete  SatVariant=Enabled  AWVariant=Passthrough  PCopyVariant=Disabled  TRVariant=Disabled  FdbkBlocksVariant=Forward  IdealPFdbkVariant=Disabled  SatFdbkVariant=Disabled  DerivativeFilterVariant=Disabled  NVariant=Disabled  NCopyVariant=Disabled_SignalSpec  FilterICVariant=Disabled  IntegratorICVariant=ExternalICs  ExternalResetVariant=ExternalReset  TRSumVariant=Passthrough  SumFdbkVariant=Disabled  SumVariant=Sum_PI
  PT1_Tustin : Subsystem  TreatAsAtomicUnit=on  SystemSampleTime=1
  Scope : Scope  NumInputPorts=4
  Scope1 : Scope  NumInputPorts=2
  Scope2 : Scope  NumInputPorts=2
  Substract Current Offset so that the linearised model works : Sum  Inputs=+-
  Substract Current Offset so that the linearised model works1 : Sum  Inputs=+-
  Substract Current Setpoint Offset : Sum  Inputs=+-
  Sum : Sum  Inputs=|+-
  Sum17 : Sum  Inputs=-+|
  Sum18 : Sum  Inputs=++|
  Switch_from_initial_Gain_to_Estimated : Switch  Criteria=u2 > Threshold
  System_Delay_Simulation : Delay  DelayLengthSource=Input port  DelayLength=600  DelayLengthUpperLimit=800  ExternalReset=Rising  SampleTime=1
      settings: InputPortMap=u0,p1,r5
  Unit Delay : UnitDelay
  Controller_Value : Outport
  wires:
  Substract Current Setpoint Offset/1 -> Sum/1
  Sum/1 -> "PID Controller P multiply 1 plus Ti "/1, Scope/1
  Hand_Mode/1 -> Get_Current_Offset/1(In1), Controller_Value/1, Substract Current Offset so that the linearised model works/1  "SmithPredictor"
  Substract Current Offset so that the linearised model works1/1 -> Scope1/2, Sum17/2
  PT1_Tustin/1(PT1_Output) -> Scope2/2, Sum18/1, System_Delay_Simulation/1
  System_Delay_Simulation/1 -> Scope1/1, Sum17/1
  Sum17/1 -> Sum18/2
  Mul_Gain_or_Estimate/1 -> Scope2/1, PT1_Tustin/1(PT1_Input)  "U"
  Switch_from_initial_Gain_to_Estimated/1 -> Mul_Gain_or_Estimate/2
  "PID Controller P multiply 1 plus Ti "/1 -> Hand_Mode/1, Scope/4
  Hand_Value/1 -> Divide/1, Hand_Mode/3
  Enable_Auto/1 -> [Enable_Auto], Hand_Mode/2
  P_Controller/1 -> Divide/2, "PID Controller P multiply 1 plus Ti "/2
  Check if Controller Integrator is 0/1 -> "PID Controller P multiply 1 plus Ti "/3
  " Dead_Time_System"/1 -> System_Delay_Simulation/2
  Gain_System/1 -> Switch_from_initial_Gain_to_Estimated/3
  Enable_Adaption/1 -> Switch_from_initial_Gain_to_Estimated/2
  EstimatedGain/1 -> Switch_from_initial_Gain_to_Estimated/1
  [Enable_Auto] -> Hand_Mode1/2
  Hand_Mode1/1 -> Mul_Gain_or_Estimate/1  "SmithPredictor"
  Constant4/1 -> Hand_Mode1/3
  [Enable_Auto] -> PT1_Tustin/5(Reset)
  [Enable_Auto] -> System_Delay_Simulation/3
  Substract Current Offset so that the linearised model works/1 -> Hand_Mode1/1
  Get_Current_Offset/1(Hold when disabled) -> Substract Current Offset so that the linearised model works/2
  [Enable_Auto] -> NOT/1
  NOT/1 -> Get_Current_Offset/Enable
  Sum18/1 -> Unit Delay/1
  Hand_Mode2/1 -> Substract Current Setpoint Offset/1
  NOT1/1 -> Get_Current_Offset1/Enable
  [Enable_Auto] -> NOT1/1
  Hand_Mode4/1 -> Substract Current Setpoint Offset/2, Substract Current Offset so that the linearised model works1/2
  Setpoint/1 -> Hand_Mode2/1
  [Enable_Auto] -> Hand_Mode2/2
  Constant2/1 -> Hand_Mode2/3
  Process_Value/1 -> Get_Current_Offset1/1(In1), Hand_Mode3/1
  [Enable_Auto] -> Hand_Mode3/2
  Constant3/1 -> Hand_Mode3/3
  Hand_Mode3/1 -> Substract Current Offset so that the linearised model works1/1
  Constant5/1 -> Hand_Mode4/3
  [Enable_Auto] -> Hand_Mode4/2
  Get_Current_Offset1/1(Hold when disabled) -> Hand_Mode4/1
  Time_Constant_System/1 -> PT1_Tustin/3(Time_Constant_System)
  Constant1/1 -> PT1_Tustin/2(Gain_System)
  Sample_Time/1 -> PT1_Tustin/4(Sample_Time)
  I_Controller/1 -> Check if Controller Integrator is 0/2, Invert Integrator/2
  Constant/1 -> Check if Controller Integrator is 0/3
  Invert Integrator/1 -> Check if Controller Integrator is 0/1
  Constant6/1 -> Invert Integrator/1
  Unit Delay/1 -> Sum/2
  [Enable_Auto] -> Scope/3, "PID Controller P multiply 1 plus Ti "/4
  Divide/1 -> "PID Controller P multiply 1 plus Ti "/5

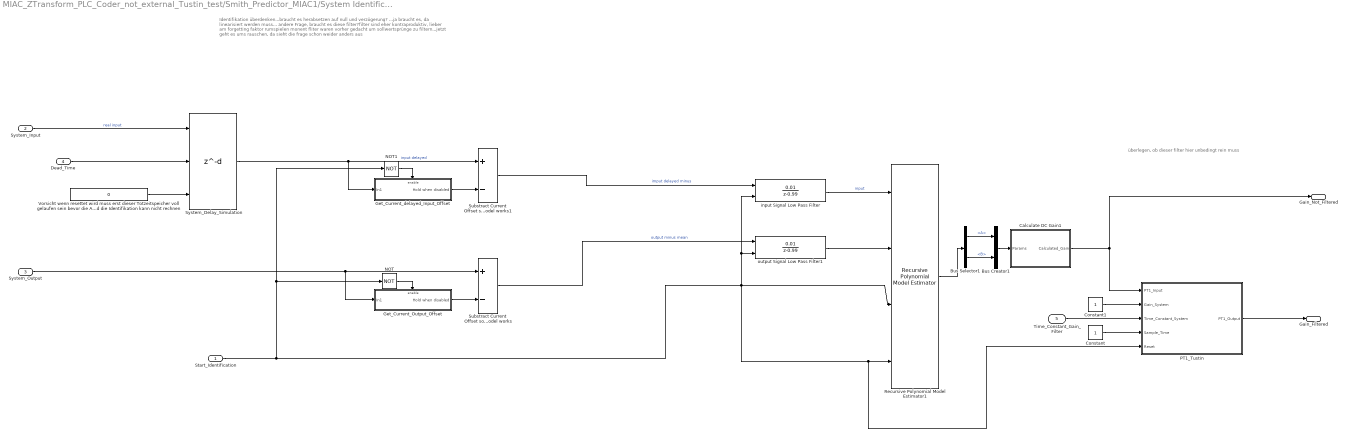
== system MIAC_ZTransform_PLC_Coder_not_external_Tustin_test/Smith_Predictor_MIAC1/System Identification ==
  note: überlegen, ob dieser filter hier unbedingt rein muss
  note: Identifikation überdenken...braucht es herabsetzen auf null und verzögerung?
      | ...ja braucht es, da linearisiert werden muss...
      |
      | andere Frage, braucht es diese filter?filter sind eher kontraproduktiv, lieber am forgetting faktor rumspielen
      | monent fliter waren vorher gedacht um sollwertsprünge zu filtern...jetzt geht es ums rauschen, da sieht die frage schon weider anders aus
  Start_Identification : Inport  SampleTime=1
  System_Input : Inport  Port=2
  System_Output : Inport  Port=3  SampleTime=1
  Dead_Time : Inport  Port=4
  Time_Constant_Gain_Filter : Inport  Port=5
  Bus Creator1 : BusCreator  Inputs=2
  Bus Selector1 : BusSelector  OutputSignals=A,B
  Calculate DC Gain1 : Subsystem  TreatAsAtomicUnit=on  SystemSampleTime=1
  Constant : Constant
  Constant1 : Constant
  Get_Current_Output_Offset : Subsystem
  Get_Current_delayed_Input_Offset : Subsystem
  NOT : Logic  Operator=NOT  IconShape=distinctive  AllPortsSameDT=off  OutDataTypeStr=boolean
  NOT1 : Logic  Operator=NOT  IconShape=distinctive  AllPortsSameDT=off  OutDataTypeStr=boolean
  PT1_Tustin : Subsystem  TreatAsAtomicUnit=on  SystemSampleTime=1
  Recursive Polynomial Model Estimator1 : slident/Estimators/Recursive Polynomial Model Estimator  ModelStructure=ARX  InitialEstimateSource=None  A0=2  B0=1  C0=1  D0=1  F0=1  nk=1  P0=10  InitialInputs=0  InitialOutputs=0  History=Infinite  WindowLength=2000  EstimationMethod=Forgetting Factor  AdaptationParameter=1  HasTimeVaryingAdaptationParameter=off  NormalizationBias=eps  OutputError=off  OutputP=off  AddEnablePort=on  ExternalReset=Rising  InputProcessing=Sample-based  Ts=1
      settings: SourceProductName=System Identification Toolbox  SourceProductBaseCode=ID
  Substract Current Offset so that the linearised model works : Sum  Inputs=+-
  Substract Current Offset so that the linearised model works1 : Sum  Inputs=+-
  System_Delay_Simulation : Delay  DelayLengthSource=Input port  DelayLength=600  DelayLengthUpperLimit=800  ExternalReset=Rising  SampleTime=1
      settings: InputPortMap=u0,p1,r5
  Vorsicht wenn resettet wird muss erst dieser Totzeitspeicher voll gelaufen sein bevor die Adaption starten darf Sonst kommt heir immer 0 raus und die Identifikation kann nicht rechnen : Constant  Value=0
  input Signal Low Pass Filter : DiscreteTransferFcn  Numerator=[0.01]  Denominator=[1 -0.99]  ExternalReset=Rising  SampleTime=1  a0EqualsOne=on
      settings: InputPortMap=u0,r7
  output Signal Low Pass Filter1 : DiscreteTransferFcn  Numerator=[0.01]  Denominator=[1 -0.99]  ExternalReset=Rising  SampleTime=1  a0EqualsOne=on
      settings: InputPortMap=u0,r7
  Gain_Filtered : Outport
  Gain_Not_Filtered : Outport  Port=2
  wires:
  Recursive Polynomial Model Estimator1/1 -> Bus Selector1/1
  input Signal Low Pass Filter/1 -> Recursive Polynomial Model Estimator1/1  "input"
  Bus Creator1/1 -> Calculate DC Gain1/1(Params)
  Bus Selector1/1 -> Bus Creator1/1  "<A>"
  Bus Selector1/2 -> Bus Creator1/2  "<B>"
  Substract Current Offset so that the linearised model works/1 -> output Signal Low Pass Filter1/1  "output minus mean"
  NOT/1 -> Get_Current_Output_Offset/Enable
  Get_Current_Output_Offset/1(Hold when disabled) -> Substract Current Offset so that the linearised model works/2
  System_Output/1 -> Get_Current_Output_Offset/1(In1), Substract Current Offset so that the linearised model works/1
  Get_Current_delayed_Input_Offset/1(Hold when disabled) -> Substract Current Offset so that the linearised model works1/2
  NOT1/1 -> Get_Current_delayed_Input_Offset/Enable
  PT1_Tustin/1(PT1_Output) -> Gain_Filtered/1
  System_Input/1 -> System_Delay_Simulation/1  "real input"
  Vorsicht wenn resettet wird muss erst dieser Totzeitspeicher voll gelaufen sein bevor die Adaption starten darf Sonst kommt heir immer 0 raus und die Identifikation kann nicht rechnen/1 -> System_Delay_Simulation/3
  Dead_Time/1 -> System_Delay_Simulation/2
  Substract Current Offset so that the linearised model works1/1 -> input Signal Low Pass Filter/1  "imput delayed minus"
  System_Delay_Simulation/1 -> Substract Current Offset so that the linearised model works1/1, Get_Current_delayed_Input_Offset/1(In1)  "input delayed"
  Calculate DC Gain1/1(Calculated_Gain) -> PT1_Tustin/1(PT1_Input), Gain_Not_Filtered/1
  Start_Identification/1 -> NOT/1, NOT1/1, PT1_Tustin/5(Reset), Recursive Polynomial Model Estimator1/4, output Signal Low Pass Filter1/2, input Signal Low Pass Filter/2, Recursive Polynomial Model Estimator1/3
  output Signal Low Pass Filter1/1 -> Recursive Polynomial Model Estimator1/2
  Constant/1 -> PT1_Tustin/4(Sample_Time)
  Constant1/1 -> PT1_Tustin/2(Gain_System)
  Time_Constant_Gain_Filter/1 -> PT1_Tustin/3(Time_Constant_System)
